simulink model "scara_env"  (R2023a)
settings: Solver=ode3  StartTime=0.0  StopTime=40  FixedStep=0.001  RelTol=1e-3  EnableMultiTasking=on
InitFcn:
  | Mp = 0.1;
  | Mc = 1;
  | l = 0.5; %half of the pole's length (distance from pivot to the center of mass of the pole)
  | g =9.81;
values from neighbouring files (symbols this model uses):
  arm_length = [2 2 2]    [script.m]
  init_pos = 10 * rand(1, num_links)'    [script.m]
  radius = 0.00002    (= 2e-05)    [script.m]
  rho = 10000000    [script.m]
settings Model: Creator=divij  LastModifiedBy=divij
settings DataIOCC: SaveFormat=Structure
settings OptimizationCC: ZeroExternalMemoryAtStartup=off  ZeroInternalMemoryAtStartup=off
settings DebuggingCC: AlgebraicLoopMsg=none
settings RTWCC: PackageGeneratedCodeAndArtifacts=on  Toolchain=Catkin  BuildConfiguration=Debug  TargetLang=C++
settings GRTTargetCC: TargetLangStandard=C++11 (ISO)  MatFileLogging=off  CodeInterfacePackaging=C++ class

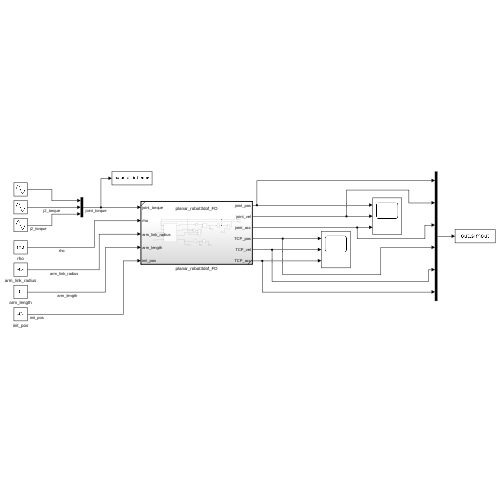
[thumbnail: Simulink's stored preview of the top-level diagram]
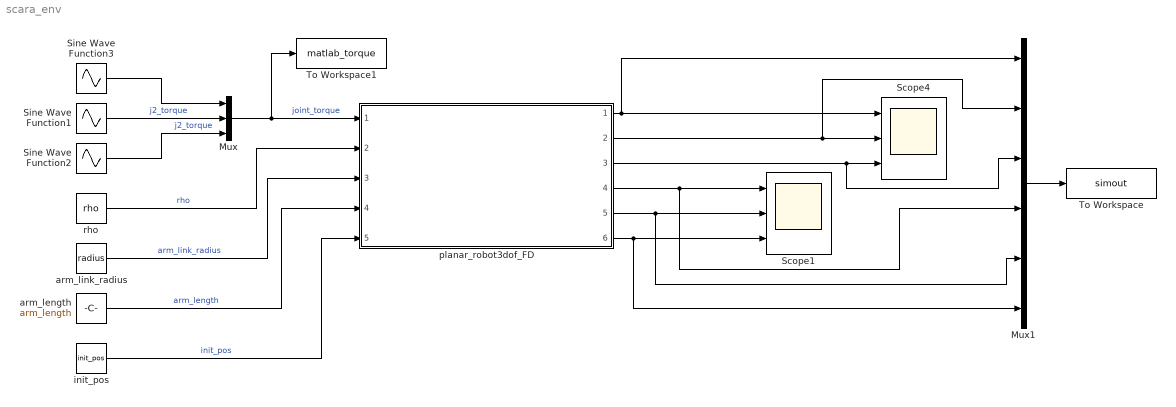
== system scara_env ==
  Mux : Mux  Inputs=3
  Mux1 : Mux  Inputs=6
  Scope1 : Scope  NumInputPorts=3
  Scope4 : Scope  NumInputPorts=3
  Sine Wave Function1 : Sin  Amplitude=2  Frequency=2  SampleTime=0
  Sine Wave Function2 : Sin  Amplitude=3  Frequency=3  SampleTime=0
  Sine Wave Function3 : Sin  SampleTime=0
  To Workspace : ToWorkspace  VariableName=simout  SaveFormat=Structure  SampleTime=-1
  To Workspace1 : ToWorkspace  VariableName=matlab_torque  SampleTime=-1
      settings: Save2DSignal=2-D array (concatenate along first dimension)
  arm_length : Constant  Value=arm_length
  arm_link_radius : Constant  Value=radius
  init_pos : Constant  Value=init_pos
  planar_robot3dof_FD : Subsystem  TreatAsAtomicUnit=on  ReferencedSubsystem=planar_robot3dof_FD
  rho : Constant  Value=rho
  wires:
  Sine Wave Function2/1 -> Mux/3  "j2_torque"
  arm_length/1 -> planar_robot3dof_FD/4  "arm_length"
  rho/1 -> planar_robot3dof_FD/2  "rho"
  planar_robot3dof_FD/3 -> Mux1/3, Scope4/3
  arm_link_radius/1 -> planar_robot3dof_FD/3  "arm_link_radius"
  Sine Wave Function3/1 -> Mux/1
  planar_robot3dof_FD/1 -> Mux1/1, Scope4/1
  Sine Wave Function1/1 -> Mux/2  "j2_torque"
  planar_robot3dof_FD/2 -> Mux1/2, Scope4/2
  Mux/1 -> planar_robot3dof_FD/1, To Workspace1/1  "joint_torque"
  planar_robot3dof_FD/5 -> Mux1/5, Scope1/2
  init_pos/1 -> planar_robot3dof_FD/5  "init_pos"
  planar_robot3dof_FD/6 -> Mux1/6, Scope1/3
  planar_robot3dof_FD/4 -> Scope1/1, Mux1/4
  Mux1/1 -> To Workspace/1
